simulink model "IEEE118_FULL_seed17_GFOL_RL_percgfor091_PyStable"  (R2023a)
(part 3 of 3)

  Line-132/RConn1 -- BUS-SG-19/RConn1 -- BUS-89/LConn1 -- Line-131/RConn1
  Line-132/RConn2 -- BUS-SG-19/RConn2 -- BUS-89/LConn2 -- Line-131/RConn2
  Line-132/RConn3 -- BUS-SG-19/RConn3 -- BUS-89/LConn3 -- Line-131/RConn3
  BUS-SG-19/LConn1 -- SG-19/RConn1
  BUS-SG-19/LConn2 -- SG-19/RConn2
  BUS-SG-19/LConn3 -- SG-19/RConn3
  Line-133/LConn1 -- BUS-89/RConn1 -- Line-134/LConn1
  Line-133/LConn2 -- BUS-89/RConn2 -- Line-134/LConn2
  Line-133/LConn3 -- BUS-89/RConn3 -- Line-134/LConn3
  Line-133/RConn1 -- BUS-Load-68/LConn1 -- BUS-90/LConn1 -- BUS-SG-20/RConn1
  Line-133/RConn2 -- BUS-Load-68/LConn2 -- BUS-90/LConn2 -- BUS-SG-20/RConn2
  Line-133/RConn3 -- BUS-Load-68/LConn3 -- BUS-90/LConn3 -- BUS-SG-20/RConn3
  BUS-Load-68/RConn1 -- Load-68/LConn1
  BUS-Load-68/RConn2 -- Load-68/LConn2
  BUS-Load-68/RConn3 -- Load-68/LConn3
  BUS-SG-20/LConn1 -- SG-20/RConn1
  BUS-SG-20/LConn2 -- SG-20/RConn2
  BUS-SG-20/LConn3 -- SG-20/RConn3
  BUS-90/RConn1 -- Line-135/LConn1
  BUS-90/RConn2 -- Line-135/LConn2
  BUS-90/RConn3 -- Line-135/LConn3
  Line-135/RConn1 -- BUS-91/LConn1
  Line-135/RConn2 -- BUS-91/LConn2
  Line-135/RConn3 -- BUS-91/LConn3
  BUS-91/RConn1 -- Line-136/LConn1
  BUS-91/RConn2 -- Line-136/LConn2
  BUS-91/RConn3 -- Line-136/LConn3
  BUS-92/LConn1 -- Line-136/RConn1 -- Line-134/RConn1
  BUS-92/LConn2 -- Line-136/RConn2 -- Line-134/RConn2
  BUS-92/LConn3 -- Line-136/RConn3 -- Line-134/RConn3
  BUS-Load-69/LConn1 -- BUS-92/RConn1 -- BUS-SG-21/RConn1 -- BUS-VSC-6/RConn1 -- BUS-VSC-16/RConn1 -- Line-137/LConn1 -- Line-140/LConn1 -- Line-139/LConn1 -- Line-138/LConn1
  BUS-Load-69/LConn2 -- BUS-92/RConn2 -- BUS-SG-21/RConn2 -- BUS-VSC-6/RConn2 -- BUS-VSC-16/RConn2 -- Line-137/LConn2 -- Line-140/LConn2 -- Line-139/LConn2 -- Line-138/LConn2
  BUS-Load-69/LConn3 -- BUS-92/RConn3 -- BUS-SG-21/RConn3 -- BUS-VSC-6/RConn3 -- BUS-VSC-16/RConn3 -- Line-137/LConn3 -- Line-140/LConn3 -- Line-139/LConn3 -- Line-138/LConn3
  BUS-Load-69/RConn1 -- Load-69/LConn1
  BUS-Load-69/RConn2 -- Load-69/LConn2
  BUS-Load-69/RConn3 -- Load-69/LConn3
  BUS-SG-21/LConn1 -- SG-21/RConn1
  BUS-SG-21/LConn2 -- SG-21/RConn2
  BUS-SG-21/LConn3 -- SG-21/RConn3
  BUS-VSC-6/LConn1 -- VSC-6/RConn1
  BUS-VSC-6/LConn2 -- VSC-6/RConn2
  BUS-VSC-6/LConn3 -- VSC-6/RConn3
  BUS-VSC-16/LConn1 -- VSC-16/RConn1
  BUS-VSC-16/LConn2 -- VSC-16/RConn2
  BUS-VSC-16/LConn3 -- VSC-16/RConn3
  BUS-93/LConn1 -- Line-137/RConn1 -- Line-141/LConn1
  BUS-93/LConn2 -- Line-137/RConn2 -- Line-141/LConn2
  BUS-93/LConn3 -- Line-137/RConn3 -- Line-141/LConn3
  BUS-93/RConn1 -- BUS-Load-70/LConn1
  BUS-93/RConn2 -- BUS-Load-70/LConn2
  BUS-93/RConn3 -- BUS-Load-70/LConn3
  BUS-Load-70/RConn1 -- Load-70/LConn1
  BUS-Load-70/RConn2 -- Load-70/LConn2
  BUS-Load-70/RConn3 -- Load-70/LConn3
  Line-141/RConn1 -- BUS-Load-71/LConn1 -- Line-142/LConn1 -- BUS-94/RConn1 -- Line-144/LConn1
  Line-141/RConn2 -- BUS-Load-71/LConn2 -- Line-142/LConn2 -- BUS-94/RConn2 -- Line-144/LConn2
  Line-141/RConn3 -- BUS-Load-71/LConn3 -- Line-142/LConn3 -- BUS-94/RConn3 -- Line-144/LConn3
  BUS-Load-71/RConn1 -- Load-71/LConn1
  BUS-Load-71/RConn2 -- Load-71/LConn2
  BUS-Load-71/RConn3 -- Load-71/LConn3
  BUS-95/LConn1 -- Line-142/RConn1 -- Line-145/LConn1
  BUS-95/LConn2 -- Line-142/RConn2 -- Line-145/LConn2
  BUS-95/LConn3 -- Line-142/RConn3 -- Line-145/LConn3
  BUS-95/RConn1 -- BUS-Load-72/LConn1
  BUS-95/RConn2 -- BUS-Load-72/LConn2
  BUS-95/RConn3 -- BUS-Load-72/LConn3
  BUS-Load-72/RConn1 -- Load-72/LConn1
  BUS-Load-72/RConn2 -- Load-72/LConn2
  BUS-Load-72/RConn3 -- Load-72/LConn3
  Line-143/LConn1 -- BUS-94/LConn1 -- Line-138/RConn1
  Line-143/LConn2 -- BUS-94/LConn2 -- Line-138/RConn2
  Line-143/LConn3 -- BUS-94/LConn3 -- Line-138/RConn3
  Line-144/RConn1 -- BUS-Load-76/LConn1 -- BUS-SG-22/RConn1 -- BUS-VSC-7/RConn1 -- Line-149/LConn1 -- Line-139/RConn1 -- Line-147/RConn1 -- BUS-100/LConn1 -- Line-148/RConn1
  Line-144/RConn2 -- BUS-Load-76/LConn2 -- BUS-SG-22/RConn2 -- BUS-VSC-7/RConn2 -- Line-149/LConn2 -- Line-139/RConn2 -- Line-147/RConn2 -- BUS-100/LConn2 -- Line-148/RConn2
  Line-144/RConn3 -- BUS-Load-76/LConn3 -- BUS-SG-22/RConn3 -- BUS-VSC-7/RConn3 -- Line-149/LConn3 -- Line-139/RConn3 -- Line-147/RConn3 -- BUS-100/LConn3 -- Line-148/RConn3
  BUS-Load-76/RConn1 -- Load-76/LConn1
  BUS-Load-76/RConn2 -- Load-76/LConn2
  BUS-Load-76/RConn3 -- Load-76/LConn3
  BUS-SG-22/LConn1 -- SG-22/RConn1
  BUS-SG-22/LConn2 -- SG-22/RConn2
  BUS-SG-22/LConn3 -- SG-22/RConn3
  BUS-VSC-7/LConn1 -- VSC-7/RConn1
  BUS-VSC-7/LConn2 -- VSC-7/RConn2
  BUS-VSC-7/LConn3 -- VSC-7/RConn3
  BUS-VSC-17/RConn1 -- BUS-100/RConn1 -- Line-150/LConn1 -- Line-152/LConn1 -- Line-151/LConn1
  BUS-VSC-17/RConn2 -- BUS-100/RConn2 -- Line-150/LConn2 -- Line-152/LConn2 -- Line-151/LConn2
  BUS-VSC-17/RConn3 -- BUS-100/RConn3 -- Line-150/LConn3 -- Line-152/LConn3 -- Line-151/LConn3
  BUS-VSC-17/LConn1 -- VSC-17/RConn1
  BUS-VSC-17/LConn2 -- VSC-17/RConn2
  BUS-VSC-17/LConn3 -- VSC-17/RConn3
  BUS-101/RConn1 -- Line-149/RConn1 -- Line-153/LConn1
  BUS-101/RConn2 -- Line-149/RConn2 -- Line-153/LConn2
  BUS-101/RConn3 -- Line-149/RConn3 -- Line-153/LConn3
  BUS-101/LConn1 -- BUS-Load-77/LConn1
  BUS-101/LConn2 -- BUS-Load-77/LConn2
  BUS-101/LConn3 -- BUS-Load-77/LConn3
  BUS-Load-77/RConn1 -- Load-77/LConn1
  BUS-Load-77/RConn2 -- Load-77/LConn2
  BUS-Load-77/RConn3 -- Load-77/LConn3
  BUS-102/LConn1 -- Line-153/RConn1 -- Line-140/RConn1
  BUS-102/LConn2 -- Line-153/RConn2 -- Line-140/RConn2
  BUS-102/LConn3 -- Line-153/RConn3 -- Line-140/RConn3
  BUS-102/RConn1 -- BUS-Load-78/LConn1
  BUS-102/RConn2 -- BUS-Load-78/LConn2
  BUS-102/RConn3 -- BUS-Load-78/LConn3
  BUS-Load-78/RConn1 -- Load-78/LConn1
  BUS-Load-78/RConn2 -- Load-78/LConn2
  BUS-Load-78/RConn3 -- Load-78/LConn3
  Line-150/RConn1 -- Line-154/LConn1 -- BUS-103/LConn1 -- Line-155/LConn1
  Line-150/RConn2 -- Line-154/LConn2 -- BUS-103/LConn2 -- Line-155/LConn2
  Line-150/RConn3 -- Line-154/LConn3 -- BUS-103/LConn3 -- Line-155/LConn3
  BUS-Load-79/LConn1 -- BUS-103/RConn1 -- Line-156/LConn1
  BUS-Load-79/LConn2 -- BUS-103/RConn2 -- Line-156/LConn2
  BUS-Load-79/LConn3 -- BUS-103/RConn3 -- Line-156/LConn3
  BUS-Load-79/RConn1 -- Load-79/LConn1
  BUS-Load-79/RConn2 -- Load-79/LConn2
  BUS-Load-79/RConn3 -- Load-79/LConn3
  Line-154/RConn1 -- BUS-Load-80/LConn1 -- BUS-104/RConn1 -- Line-157/LConn1
  Line-154/RConn2 -- BUS-Load-80/LConn2 -- BUS-104/RConn2 -- Line-157/LConn2
  Line-154/RConn3 -- BUS-Load-80/LConn3 -- BUS-104/RConn3 -- Line-157/LConn3
  BUS-Load-80/RConn1 -- Load-80/LConn1
  BUS-Load-80/RConn2 -- Load-80/LConn2
  BUS-Load-80/RConn3 -- Load-80/LConn3
  Line-157/RConn1 -- BUS-VSC-18/RConn1 -- Line-158/LConn1 -- BUS-105/LConn1 -- Line-159/LConn1
  Line-157/RConn2 -- BUS-VSC-18/RConn2 -- Line-158/LConn2 -- BUS-105/LConn2 -- Line-159/LConn2
  Line-157/RConn3 -- BUS-VSC-18/RConn3 -- Line-158/LConn3 -- BUS-105/LConn3 -- Line-159/LConn3
  BUS-Load-81/LConn1 -- BUS-105/RConn1 -- BUS-SG-23/RConn1 -- BUS-VSC-8/RConn1 -- Line-160/LConn1 -- Line-155/RConn1
  BUS-Load-81/LConn2 -- BUS-105/RConn2 -- BUS-SG-23/RConn2 -- BUS-VSC-8/RConn2 -- Line-160/LConn2 -- Line-155/RConn2
  BUS-Load-81/LConn3 -- BUS-105/RConn3 -- BUS-SG-23/RConn3 -- BUS-VSC-8/RConn3 -- Line-160/LConn3 -- Line-155/RConn3
  BUS-Load-81/RConn1 -- Load-81/LConn1
  BUS-Load-81/RConn2 -- Load-81/LConn2
  BUS-Load-81/RConn3 -- Load-81/LConn3
  BUS-SG-23/LConn1 -- SG-23/RConn1
  BUS-SG-23/LConn2 -- SG-23/RConn2
  BUS-SG-23/LConn3 -- SG-23/RConn3
  BUS-VSC-8/LConn1 -- VSC-8/RConn1
  BUS-VSC-8/LConn2 -- VSC-8/RConn2
  BUS-VSC-8/LConn3 -- VSC-8/RConn3
  BUS-VSC-18/LConn1 -- VSC-18/RConn1
  BUS-VSC-18/LConn2 -- VSC-18/RConn2
  BUS-VSC-18/LConn3 -- VSC-18/RConn3
  BUS-106/RConn1 -- Line-158/RConn1 -- Line-161/LConn1
  BUS-106/RConn2 -- Line-158/RConn2 -- Line-161/LConn2
  BUS-106/RConn3 -- Line-158/RConn3 -- Line-161/LConn3
  BUS-Load-82/LConn1 -- BUS-106/LConn1 -- Line-152/RConn1
  BUS-Load-82/LConn2 -- BUS-106/LConn2 -- Line-152/RConn2
  BUS-Load-82/LConn3 -- BUS-106/LConn3 -- Line-152/RConn3
  BUS-Load-82/RConn1 -- Load-82/LConn1
  BUS-Load-82/RConn2 -- Load-82/LConn2
  BUS-Load-82/RConn3 -- Load-82/LConn3
  Line-161/RConn1 -- BUS-Load-83/LConn1 -- BUS-107/LConn1 -- BUS-SG-24/RConn1
  Line-161/RConn2 -- BUS-Load-83/LConn2 -- BUS-107/LConn2 -- BUS-SG-24/RConn2
  Line-161/RConn3 -- BUS-Load-83/LConn3 -- BUS-107/LConn3 -- BUS-SG-24/RConn3
  BUS-Load-83/RConn1 -- Load-83/LConn1
  BUS-Load-83/RConn2 -- Load-83/LConn2
  BUS-Load-83/RConn3 -- Load-83/LConn3
  BUS-SG-24/LConn1 -- SG-24/RConn1
  BUS-SG-24/LConn2 -- SG-24/RConn2
  BUS-SG-24/LConn3 -- SG-24/RConn3
  Line-159/RConn1 -- BUS-107/RConn1
  Line-159/RConn2 -- BUS-107/RConn2
  Line-159/RConn3 -- BUS-107/RConn3
  Line-160/RConn1 -- BUS-108/LConn1
  Line-160/RConn2 -- BUS-108/LConn2
  Line-160/RConn3 -- BUS-108/LConn3
  BUS-Load-84/LConn1 -- BUS-108/RConn1 -- Line-162/LConn1
  BUS-Load-84/LConn2 -- BUS-108/RConn2 -- Line-162/LConn2
  BUS-Load-84/LConn3 -- BUS-108/RConn3 -- Line-162/LConn3
  BUS-Load-84/RConn1 -- Load-84/LConn1
  BUS-Load-84/RConn2 -- Load-84/LConn2
  BUS-Load-84/RConn3 -- Load-84/LConn3
  Line-162/RConn1 -- BUS-109/LConn1
  Line-162/RConn2 -- BUS-109/LConn2
  Line-162/RConn3 -- BUS-109/LConn3
  BUS-Load-85/LConn1 -- BUS-109/RConn1 -- Line-163/LConn1
  BUS-Load-85/LConn2 -- BUS-109/RConn2 -- Line-163/LConn2
  BUS-Load-85/LConn3 -- BUS-109/RConn3 -- Line-163/LConn3
  BUS-Load-85/RConn1 -- Load-85/LConn1
  BUS-Load-85/RConn2 -- Load-85/LConn2
  BUS-Load-85/RConn3 -- Load-85/LConn3
  BUS-110/LConn1 -- Line-163/RConn1 -- Line-156/RConn1
  BUS-110/LConn2 -- Line-163/RConn2 -- Line-156/RConn2
  BUS-110/LConn3 -- Line-163/RConn3 -- Line-156/RConn3
  BUS-Load-86/LConn1 -- BUS-110/RConn1 -- BUS-VSC-9/RConn1 -- BUS-VSC-19/RConn1 -- Line-164/LConn1
  BUS-Load-86/LConn2 -- BUS-110/RConn2 -- BUS-VSC-9/RConn2 -- BUS-VSC-19/RConn2 -- Line-164/LConn2
  BUS-Load-86/LConn3 -- BUS-110/RConn3 -- BUS-VSC-9/RConn3 -- BUS-VSC-19/RConn3 -- Line-164/LConn3
  BUS-Load-86/RConn1 -- Load-86/LConn1
  BUS-Load-86/RConn2 -- Load-86/LConn2
  BUS-Load-86/RConn3 -- Load-86/LConn3
  BUS-VSC-9/LConn1 -- VSC-9/RConn1
  BUS-VSC-9/LConn2 -- VSC-9/RConn2
  BUS-VSC-9/LConn3 -- VSC-9/RConn3
  BUS-VSC-19/LConn1 -- VSC-19/RConn1
  BUS-VSC-19/LConn2 -- VSC-19/RConn2
  BUS-VSC-19/LConn3 -- VSC-19/RConn3
  Line-164/RConn1 -- BUS-112/LConn1
  Line-164/RConn2 -- BUS-112/LConn2
  Line-164/RConn3 -- BUS-112/LConn3
  BUS-Load-87/LConn1 -- BUS-112/RConn1 -- BUS-SG-25/RConn1 -- BUS-VSC-10/RConn1 -- BUS-VSC-20/RConn1
  BUS-Load-87/LConn2 -- BUS-112/RConn2 -- BUS-SG-25/RConn2 -- BUS-VSC-10/RConn2 -- BUS-VSC-20/RConn2
  BUS-Load-87/LConn3 -- BUS-112/RConn3 -- BUS-SG-25/RConn3 -- BUS-VSC-10/RConn3 -- BUS-VSC-20/RConn3
  BUS-Load-87/RConn1 -- Load-87/LConn1
  BUS-Load-87/RConn2 -- Load-87/LConn2
  BUS-Load-87/RConn3 -- Load-87/LConn3
  BUS-SG-25/LConn1 -- SG-25/RConn1
  BUS-SG-25/LConn2 -- SG-25/RConn2
  BUS-SG-25/LConn3 -- SG-25/RConn3
  BUS-VSC-10/LConn1 -- VSC-10/RConn1
  BUS-VSC-10/LConn2 -- VSC-10/RConn2
  BUS-VSC-10/LConn3 -- VSC-10/RConn3
  BUS-VSC-20/LConn1 -- VSC-20/RConn1
  BUS-VSC-20/LConn2 -- VSC-20/RConn2
  BUS-VSC-20/LConn3 -- VSC-20/RConn3
  Line-151/RConn1 -- BUS-104/LConn1
  Line-151/RConn2 -- BUS-104/LConn2
  Line-151/RConn3 -- BUS-104/LConn3
  BUS-98/RConn1 -- Line-147/LConn1
  BUS-98/RConn2 -- Line-147/LConn2
  BUS-98/RConn3 -- Line-147/LConn3
  BUS-Load-75/LConn1 -- BUS-98/LConn1 -- Line-122/RConn1
  BUS-Load-75/LConn2 -- BUS-98/LConn2 -- Line-122/RConn2
  BUS-Load-75/LConn3 -- BUS-98/LConn3 -- Line-122/RConn3
  BUS-Load-75/RConn1 -- Load-75/LConn1
  BUS-Load-75/RConn2 -- Load-75/LConn2
  BUS-Load-75/RConn3 -- Load-75/LConn3
  BUS-99/RConn1 -- Line-148/LConn1
  BUS-99/RConn2 -- Line-148/LConn2
  BUS-99/RConn3 -- Line-148/LConn3
  Line-123/RConn1 -- BUS-99/LConn1
  Line-123/RConn2 -- BUS-99/LConn2
  Line-123/RConn3 -- BUS-99/LConn3
  Line-117/LConn1 -- BUS-77/LConn1 -- BUS-Load-58/LConn1 -- BUS-SG-16/RConn1 -- Line-115/LConn1 -- Line-113/RConn1
  Line-117/LConn2 -- BUS-77/LConn2 -- BUS-Load-58/LConn2 -- BUS-SG-16/RConn2 -- Line-115/LConn2 -- Line-113/RConn2
  Line-117/LConn3 -- BUS-77/LConn3 -- BUS-Load-58/LConn3 -- BUS-SG-16/RConn3 -- Line-115/LConn3 -- Line-113/RConn3
  BUS-Load-58/RConn1 -- Load-58/LConn1
  BUS-Load-58/RConn2 -- Load-58/LConn2
  BUS-Load-58/RConn3 -- Load-58/LConn3
  BUS-SG-16/LConn1 -- SG-16/RConn1
  BUS-SG-16/LConn2 -- SG-16/RConn2
  BUS-SG-16/LConn3 -- SG-16/RConn3
  BUS-78/RConn1 -- Line-115/RConn1 -- Line-118/LConn1
  BUS-78/RConn2 -- Line-115/RConn2 -- Line-118/LConn2
  BUS-78/RConn3 -- Line-115/RConn3 -- Line-118/LConn3
  BUS-78/LConn1 -- BUS-Load-59/LConn1
  BUS-78/LConn2 -- BUS-Load-59/LConn2
  BUS-78/LConn3 -- BUS-Load-59/LConn3
  BUS-Load-59/RConn1 -- Load-59/LConn1
  BUS-Load-59/RConn2 -- Load-59/LConn2
  BUS-Load-59/RConn3 -- Load-59/LConn3
  BUS-79/LConn1 -- Line-118/RConn1 -- BUS-Load-60/LConn1
  BUS-79/LConn2 -- Line-118/RConn2 -- BUS-Load-60/LConn2
  BUS-79/LConn3 -- Line-118/RConn3 -- BUS-Load-60/LConn3
  BUS-Load-60/RConn1 -- Load-60/LConn1
  BUS-Load-60/RConn2 -- Load-60/LConn2
  BUS-Load-60/RConn3 -- Load-60/LConn3
  BUS-79/RConn1 -- Line-119/LConn1
  BUS-79/RConn2 -- Line-119/LConn2
  BUS-79/RConn3 -- Line-119/LConn3
  Line-116/LConn1 -- BUS-77/RConn1 -- Line-104/RConn1 -- Line-111/RConn1
  Line-116/LConn2 -- BUS-77/RConn2 -- Line-104/RConn2 -- Line-111/RConn2
  Line-116/LConn3 -- BUS-77/RConn3 -- Line-104/RConn3 -- Line-111/RConn3
  Line-104/LConn1 -- BUS-69/LConn1 -- Line-103/LConn1
  Line-104/LConn2 -- BUS-69/LConn2 -- Line-103/LConn2
  Line-104/LConn3 -- BUS-69/LConn3 -- Line-103/LConn3
  Line-102/LConn1 -- BUS-69/RConn1 -- Line-76/RConn1 -- Line-70/RConn1 -- Line-173/RConn1
  Line-102/LConn2 -- BUS-69/RConn2 -- Line-76/RConn2 -- Line-70/RConn2 -- Line-173/RConn2
  Line-102/LConn3 -- BUS-69/RConn3 -- Line-76/RConn3 -- Line-70/RConn3 -- Line-173/RConn3
  Line-102/RConn1 -- Line-105/LConn1 -- Line-106/LConn1 -- BUS-70/LConn1 -- Line-107/LConn1
  Line-102/RConn2 -- Line-105/LConn2 -- Line-106/LConn2 -- BUS-70/LConn2 -- Line-107/LConn2
  Line-102/RConn3 -- Line-105/LConn3 -- Line-106/LConn3 -- BUS-70/LConn3 -- Line-107/LConn3
  BUS-Load-54/LConn1 -- BUS-70/RConn1 -- BUS-SG-12/RConn1 -- Line-36/RConn1
  BUS-Load-54/LConn2 -- BUS-70/RConn2 -- BUS-SG-12/RConn2 -- Line-36/RConn2
  BUS-Load-54/LConn3 -- BUS-70/RConn3 -- BUS-SG-12/RConn3 -- Line-36/RConn3
  BUS-Load-54/RConn1 -- Load-54/LConn1
  BUS-Load-54/RConn2 -- Load-54/LConn2
  BUS-Load-54/RConn3 -- Load-54/LConn3
  BUS-SG-12/LConn1 -- SG-12/RConn1
  BUS-SG-12/LConn2 -- SG-12/RConn2
  BUS-SG-12/LConn3 -- SG-12/RConn3
  BUS-71/RConn1 -- Line-105/RConn1 -- Line-108/LConn1
  BUS-71/RConn2 -- Line-105/RConn2 -- Line-108/LConn2
  BUS-71/RConn3 -- Line-105/RConn3 -- Line-108/LConn3
  Line-108/RConn1 -- BUS-72/LConn1
  Line-108/RConn2 -- BUS-72/LConn2
  Line-108/RConn3 -- BUS-72/LConn3
  BUS-SG-13/RConn1 -- BUS-72/RConn1 -- Line-37/RConn1
  BUS-SG-13/RConn2 -- BUS-72/RConn2 -- Line-37/RConn2
  BUS-SG-13/RConn3 -- BUS-72/RConn3 -- Line-37/RConn3
  BUS-SG-13/LConn1 -- SG-13/RConn1
  BUS-SG-13/LConn2 -- SG-13/RConn2
  BUS-SG-13/LConn3 -- SG-13/RConn3
  Line-37/LConn1 -- BUS-24/LConn1 -- Line-36/LConn1
  Line-37/LConn2 -- BUS-24/LConn2 -- Line-36/LConn2
  Line-37/LConn3 -- BUS-24/LConn3 -- Line-36/LConn3
  Line-33/LConn1 -- BUS-23/LConn1 -- BUS-Load-19/LConn1
  Line-33/LConn2 -- BUS-23/LConn2 -- BUS-Load-19/LConn2
  Line-33/LConn3 -- BUS-23/LConn3 -- BUS-Load-19/LConn3
  Line-33/RConn1 -- BUS-24/RConn1
  Line-33/RConn2 -- BUS-24/RConn2
  Line-33/RConn3 -- BUS-24/RConn3
  BUS-Load-19/RConn1 -- Load-19/LConn1
  BUS-Load-19/RConn2 -- Load-19/LConn2
  BUS-Load-19/RConn3 -- Load-19/LConn3
  Line-34/LConn1 -- BUS-23/RConn1 -- Line-32/RConn1 -- Line-35/LConn1
  Line-34/LConn2 -- BUS-23/RConn2 -- Line-32/RConn2 -- Line-35/LConn2
  Line-34/LConn3 -- BUS-23/RConn3 -- Line-32/RConn3 -- Line-35/LConn3
  Line-34/RConn1 -- BUS-25/LConn1
  Line-34/RConn2 -- BUS-25/LConn2
  Line-34/RConn3 -- BUS-25/LConn3
  Line-38/LConn1 -- BUS-25/RConn1 -- Line-168/LConn1
  Line-38/LConn2 -- BUS-25/RConn2 -- Line-168/LConn2
  Line-38/LConn3 -- BUS-25/RConn3 -- Line-168/LConn3
  Line-38/RConn1 -- BUS-Load-20/LConn1 -- BUS-27/LConn1 -- Line-41/LConn1
  Line-38/RConn2 -- BUS-Load-20/LConn2 -- BUS-27/LConn2 -- Line-41/LConn2
  Line-38/RConn3 -- BUS-Load-20/LConn3 -- BUS-27/LConn3 -- Line-41/LConn3
  BUS-Load-20/RConn1 -- Load-20/LConn1
  BUS-Load-20/RConn2 -- Load-20/LConn2
  BUS-Load-20/RConn3 -- Load-20/LConn3
  Line-40/LConn1 -- BUS-27/RConn1 -- Line-42/LConn1
  Line-40/LConn2 -- BUS-27/RConn2 -- Line-42/LConn2
  Line-40/LConn3 -- BUS-27/RConn3 -- Line-42/LConn3
  Line-40/RConn1 -- BUS-28/LConn1
  Line-40/RConn2 -- BUS-28/LConn2
  Line-40/RConn3 -- BUS-28/LConn3
  BUS-Load-21/LConn1 -- BUS-28/RConn1 -- Line-43/LConn1
  BUS-Load-21/LConn2 -- BUS-28/RConn2 -- Line-43/LConn2
  BUS-Load-21/LConn3 -- BUS-28/RConn3 -- Line-43/LConn3
  BUS-Load-21/RConn1 -- Load-21/LConn1
  BUS-Load-21/RConn2 -- Load-21/LConn2
  BUS-Load-21/RConn3 -- Load-21/LConn3
  BUS-29/LConn1 -- Line-43/RConn1 -- Line-44/LConn1
  BUS-29/LConn2 -- Line-43/RConn2 -- Line-44/LConn2
  BUS-29/LConn3 -- Line-43/RConn3 -- Line-44/LConn3
  BUS-29/RConn1 -- BUS-Load-22/LConn1
  BUS-29/RConn2 -- BUS-Load-22/LConn2
  BUS-29/RConn3 -- BUS-Load-22/LConn3
  BUS-Load-22/RConn1 -- Load-22/LConn1
  BUS-Load-22/RConn2 -- Load-22/LConn2
  BUS-Load-22/RConn3 -- Load-22/LConn3
  Line-44/RConn1 -- BUS-VSC-2/RConn1 -- BUS-VSC-12/RConn1 -- BUS-31/RConn1 -- Line-25/RConn1
  Line-44/RConn2 -- BUS-VSC-2/RConn2 -- BUS-VSC-12/RConn2 -- BUS-31/RConn2 -- Line-25/RConn2
  Line-44/RConn3 -- BUS-VSC-2/RConn3 -- BUS-VSC-12/RConn3 -- BUS-31/RConn3 -- Line-25/RConn3
  BUS-Load-23/LConn1 -- BUS-31/LConn1 -- Line-46/LConn1
  BUS-Load-23/LConn2 -- BUS-31/LConn2 -- Line-46/LConn2
  BUS-Load-23/LConn3 -- BUS-31/LConn3 -- Line-46/LConn3
  BUS-Load-23/RConn1 -- Load-23/LConn1
  BUS-Load-23/RConn2 -- Load-23/LConn2
  BUS-Load-23/RConn3 -- Load-23/LConn3
  BUS-VSC-2/LConn1 -- VSC-2/RConn1
  BUS-VSC-2/LConn2 -- VSC-2/RConn2
  BUS-VSC-2/LConn3 -- VSC-2/RConn3
  BUS-VSC-12/LConn1 -- VSC-12/RConn1
  BUS-VSC-12/LConn2 -- VSC-12/RConn2
  BUS-VSC-12/LConn3 -- VSC-12/RConn3
  Line-46/RConn1 -- BUS-VSC-3/RConn1 -- Line-47/LConn1 -- Line-48/LConn1 -- BUS-32/RConn1 -- Line-41/RConn1
  Line-46/RConn2 -- BUS-VSC-3/RConn2 -- Line-47/LConn2 -- Line-48/LConn2 -- BUS-32/RConn2 -- Line-41/RConn2
  Line-46/RConn3 -- BUS-VSC-3/RConn3 -- Line-47/LConn3 -- Line-48/LConn3 -- BUS-32/RConn3 -- Line-41/RConn3
  BUS-Load-24/LConn1 -- BUS-32/LConn1 -- BUS-SG-3/RConn1 -- BUS-VSC-13/RConn1 -- Line-35/RConn1
  BUS-Load-24/LConn2 -- BUS-32/LConn2 -- BUS-SG-3/RConn2 -- BUS-VSC-13/RConn2 -- Line-35/RConn2
  BUS-Load-24/LConn3 -- BUS-32/LConn3 -- BUS-SG-3/RConn3 -- BUS-VSC-13/RConn3 -- Line-35/RConn3
  BUS-Load-24/RConn1 -- Load-24/LConn1
  BUS-Load-24/RConn2 -- Load-24/LConn2
  BUS-Load-24/RConn3 -- Load-24/LConn3
  BUS-SG-3/LConn1 -- SG-3/RConn1
  BUS-SG-3/LConn2 -- SG-3/RConn2
  BUS-SG-3/LConn3 -- SG-3/RConn3
  BUS-VSC-3/LConn1 -- VSC-3/RConn1
  BUS-VSC-3/LConn2 -- VSC-3/RConn2
  BUS-VSC-3/LConn3 -- VSC-3/RConn3
  BUS-VSC-13/LConn1 -- VSC-13/RConn1
  BUS-VSC-13/LConn2 -- VSC-13/RConn2
  BUS-VSC-13/LConn3 -- VSC-13/RConn3
  BUS-113/LConn1 -- Line-47/RConn1 -- BUS-SG-26/RConn1
  BUS-113/LConn2 -- Line-47/RConn2 -- BUS-SG-26/RConn2
  BUS-113/LConn3 -- Line-47/RConn3 -- BUS-SG-26/RConn3
  BUS-SG-26/LConn1 -- SG-26/RConn1
  BUS-SG-26/LConn2 -- SG-26/RConn2
  BUS-SG-26/LConn3 -- SG-26/RConn3
  Line-26/LConn1 -- BUS-17/LConn1 -- Line-167/LConn1 -- Line-25/LConn1
  Line-26/LConn2 -- BUS-17/LConn2 -- Line-167/LConn2 -- Line-25/LConn2
  Line-26/LConn3 -- BUS-17/LConn3 -- Line-167/LConn3 -- Line-25/LConn3
  Line-26/RConn1 -- BUS-113/RConn1
  Line-26/RConn2 -- BUS-113/RConn2
  Line-26/RConn3 -- BUS-113/RConn3
  BUS-Load-13/LConn1 -- BUS-17/RConn1 -- Line-24/LConn1 -- Line-20/RConn1 -- Line-23/RConn1
  BUS-Load-13/LConn2 -- BUS-17/RConn2 -- Line-24/LConn2 -- Line-20/RConn2 -- Line-23/RConn2
  BUS-Load-13/LConn3 -- BUS-17/RConn3 -- Line-24/LConn3 -- Line-20/RConn3 -- Line-23/RConn3
  BUS-Load-13/RConn1 -- Load-13/LConn1
  BUS-Load-13/RConn2 -- Load-13/LConn2
  BUS-Load-13/RConn3 -- Load-13/LConn3
  BUS-18/LConn1 -- Line-24/RConn1 -- BUS-Load-14/LConn1
  BUS-18/LConn2 -- Line-24/RConn2 -- BUS-Load-14/LConn2
  BUS-18/LConn3 -- Line-24/RConn3 -- BUS-Load-14/LConn3
  BUS-Load-14/RConn1 -- Load-14/LConn1
  BUS-Load-14/RConn2 -- Load-14/LConn2
  BUS-Load-14/RConn3 -- Load-14/LConn3
  BUS-18/RConn1 -- Line-27/LConn1
  BUS-18/RConn2 -- Line-27/LConn2
  BUS-18/RConn3 -- Line-27/LConn3
  Line-27/RConn1 -- Line-28/LConn1 -- BUS-19/LConn1 -- Line-29/LConn1
  Line-27/RConn2 -- Line-28/LConn2 -- BUS-19/LConn2 -- Line-29/LConn2
  Line-27/RConn3 -- Line-28/LConn3 -- BUS-19/LConn3 -- Line-29/LConn3
  BUS-Load-15/LConn1 -- BUS-19/RConn1 -- BUS-SG-2/RConn1 -- BUS-VSC-1/RConn1 -- BUS-VSC-11/RConn1 -- Line-21/RConn1
  BUS-Load-15/LConn2 -- BUS-19/RConn2 -- BUS-SG-2/RConn2 -- BUS-VSC-1/RConn2 -- BUS-VSC-11/RConn2 -- Line-21/RConn2
  BUS-Load-15/LConn3 -- BUS-19/RConn3 -- BUS-SG-2/RConn3 -- BUS-VSC-1/RConn3 -- BUS-VSC-11/RConn3 -- Line-21/RConn3
  BUS-Load-15/RConn1 -- Load-15/LConn1
  BUS-Load-15/RConn2 -- Load-15/LConn2
  BUS-Load-15/RConn3 -- Load-15/LConn3
  BUS-SG-2/LConn1 -- SG-2/RConn1
  BUS-SG-2/LConn2 -- SG-2/RConn2
  BUS-SG-2/LConn3 -- SG-2/RConn3
  BUS-VSC-1/LConn1 -- VSC-1/RConn1
  BUS-VSC-1/LConn2 -- VSC-1/RConn2
  BUS-VSC-1/LConn3 -- VSC-1/RConn3
  BUS-VSC-11/LConn1 -- VSC-11/RConn1
  BUS-VSC-11/LConn2 -- VSC-11/RConn2
  BUS-VSC-11/LConn3 -- VSC-11/RConn3
  BUS-20/RConn1 -- Line-28/RConn1 -- BUS-Load-16/LConn1
  BUS-20/RConn2 -- Line-28/RConn2 -- BUS-Load-16/LConn2
  BUS-20/RConn3 -- Line-28/RConn3 -- BUS-Load-16/LConn3
  BUS-Load-16/RConn1 -- Load-16/LConn1
  BUS-Load-16/RConn2 -- Load-16/LConn2
  BUS-Load-16/RConn3 -- Load-16/LConn3
  BUS-20/LConn1 -- Line-30/LConn1
  BUS-20/LConn2 -- Line-30/LConn2
  BUS-20/LConn3 -- Line-30/LConn3
  BUS-21/RConn1 -- Line-30/RConn1 -- BUS-Load-17/LConn1
  BUS-21/RConn2 -- Line-30/RConn2 -- BUS-Load-17/LConn2
  BUS-21/RConn3 -- Line-30/RConn3 -- BUS-Load-17/LConn3
  BUS-Load-17/RConn1 -- Load-17/LConn1
  BUS-Load-17/RConn2 -- Load-17/LConn2
  BUS-Load-17/RConn3 -- Load-17/LConn3
  BUS-21/LConn1 -- Line-31/LConn1
  BUS-21/LConn2 -- Line-31/LConn2
  BUS-21/LConn3 -- Line-31/LConn3
  Line-31/RConn1 -- BUS-22/RConn1
  Line-31/RConn2 -- BUS-22/RConn2
  Line-31/RConn3 -- BUS-22/RConn3
  BUS-Load-18/LConn1 -- BUS-22/LConn1 -- Line-32/LConn1
  BUS-Load-18/LConn2 -- BUS-22/LConn2 -- Line-32/LConn2
  BUS-Load-18/LConn3 -- BUS-22/LConn3 -- Line-32/LConn3
  BUS-Load-18/RConn1 -- Load-18/LConn1
  BUS-Load-18/RConn2 -- Load-18/LConn2
  BUS-Load-18/RConn3 -- Load-18/LConn3
  Line-29/RConn1 -- BUS-Load-26/LConn1 -- BUS-SG-4/RConn1 -- BUS-34/RConn1 -- Line-50/LConn1
  Line-29/RConn2 -- BUS-Load-26/LConn2 -- BUS-SG-4/RConn2 -- BUS-34/RConn2 -- Line-50/LConn2
  Line-29/RConn3 -- BUS-Load-26/LConn3 -- BUS-SG-4/RConn3 -- BUS-34/RConn3 -- Line-50/LConn3
  BUS-Load-26/RConn1 -- Load-26/LConn1
  BUS-Load-26/RConn2 -- Load-26/LConn2
  BUS-Load-26/RConn3 -- Load-26/LConn3
  BUS-SG-4/LConn1 -- SG-4/RConn1
  BUS-SG-4/LConn2 -- SG-4/RConn2
  BUS-SG-4/LConn3 -- SG-4/RConn3
  BUS-36/LConn1 -- Line-50/RConn1 -- Line-53/RConn1
  BUS-36/LConn2 -- Line-50/RConn2 -- Line-53/RConn2
  BUS-36/LConn3 -- Line-50/RConn3 -- Line-53/RConn3
  BUS-Load-28/LConn1 -- BUS-36/RConn1 -- BUS-SG-5/RConn1
  BUS-Load-28/LConn2 -- BUS-36/RConn2 -- BUS-SG-5/RConn2
  BUS-Load-28/LConn3 -- BUS-36/RConn3 -- BUS-SG-5/RConn3
  BUS-Load-28/RConn1 -- Load-28/LConn1
  BUS-Load-28/RConn2 -- Load-28/LConn2
  BUS-Load-28/RConn3 -- Load-28/LConn3
  BUS-SG-5/LConn1 -- SG-5/RConn1
  BUS-SG-5/LConn2 -- SG-5/RConn2
  BUS-SG-5/LConn3 -- SG-5/RConn3
  Line-53/LConn1 -- BUS-35/RConn1 -- BUS-Load-27/LConn1
  Line-53/LConn2 -- BUS-35/RConn2 -- BUS-Load-27/LConn2
  Line-53/LConn3 -- BUS-35/RConn3 -- BUS-Load-27/LConn3
  BUS-Load-27/RConn1 -- Load-27/LConn1
  BUS-Load-27/RConn2 -- Load-27/LConn2
  BUS-Load-27/RConn3 -- Load-27/LConn3
  BUS-35/LConn1 -- Line-54/LConn1
  BUS-35/LConn2 -- Line-54/LConn2
  BUS-35/LConn3 -- Line-54/LConn3
  Line-54/RConn1 -- BUS-Load-29/LConn1 -- Line-49/RConn1 -- BUS-37/RConn1 -- Line-51/RConn1
  Line-54/RConn2 -- BUS-Load-29/LConn2 -- Line-49/RConn2 -- BUS-37/RConn2 -- Line-51/RConn2
  Line-54/RConn3 -- BUS-Load-29/LConn3 -- Line-49/RConn3 -- BUS-37/RConn3 -- Line-51/RConn3
  BUS-Load-29/RConn1 -- Load-29/LConn1
  BUS-Load-29/RConn2 -- Load-29/LConn2
  BUS-Load-29/RConn3 -- Load-29/LConn3
  Line-55/LConn1 -- BUS-37/LConn1 -- Line-56/LConn1 -- Line-169/LConn1
  Line-55/LConn2 -- BUS-37/LConn2 -- Line-56/LConn2 -- Line-169/LConn2
  Line-55/LConn3 -- BUS-37/LConn3 -- Line-56/LConn3 -- Line-169/LConn3
  Line-55/RConn1 -- BUS-39/RConn1
  Line-55/RConn2 -- BUS-39/RConn2
  Line-55/RConn3 -- BUS-39/RConn3
  BUS-39/LConn1 -- Line-58/LConn1
  BUS-39/LConn2 -- Line-58/LConn2
  BUS-39/LConn3 -- Line-58/LConn3
  Line-58/RConn1 -- BUS-Load-30/LConn1 -- BUS-SG-6/RConn1 -- BUS-40/RConn1 -- Line-56/RConn1
  Line-58/RConn2 -- BUS-Load-30/LConn2 -- BUS-SG-6/RConn2 -- BUS-40/RConn2 -- Line-56/RConn2
  Line-58/RConn3 -- BUS-Load-30/LConn3 -- BUS-SG-6/RConn3 -- BUS-40/RConn3 -- Line-56/RConn3
  BUS-Load-30/RConn1 -- Load-30/LConn1
  BUS-Load-30/RConn2 -- Load-30/LConn2
  BUS-Load-30/RConn3 -- Load-30/LConn3
  BUS-SG-6/LConn1 -- SG-6/RConn1
  BUS-SG-6/LConn2 -- SG-6/RConn2
  BUS-SG-6/LConn3 -- SG-6/RConn3
  Line-59/LConn1 -- BUS-40/LConn1 -- Line-60/LConn1
  Line-59/LConn2 -- BUS-40/LConn2 -- Line-60/LConn2
  Line-59/LConn3 -- BUS-40/LConn3 -- Line-60/LConn3
  BUS-41/RConn1 -- Line-59/RConn1 -- BUS-Load-31/LConn1
  BUS-41/RConn2 -- Line-59/RConn2 -- BUS-Load-31/LConn2
  BUS-41/RConn3 -- Line-59/RConn3 -- BUS-Load-31/LConn3
  BUS-Load-31/RConn1 -- Load-31/LConn1
  BUS-Load-31/RConn2 -- Load-31/LConn2
  BUS-Load-31/RConn3 -- Load-31/LConn3
  BUS-41/LConn1 -- Line-61/LConn1
  BUS-41/LConn2 -- Line-61/LConn2
  BUS-41/LConn3 -- Line-61/LConn3
  Line-61/RConn1 -- BUS-Load-32/LConn1 -- BUS-42/RConn1 -- Line-60/RConn1
  Line-61/RConn2 -- BUS-Load-32/LConn2 -- BUS-42/RConn2 -- Line-60/RConn2
  Line-61/RConn3 -- BUS-Load-32/LConn3 -- BUS-42/RConn3 -- Line-60/RConn3
  BUS-Load-32/RConn1 -- Load-32/LConn1
  BUS-Load-32/RConn2 -- Load-32/LConn2
  BUS-Load-32/RConn3 -- Load-32/LConn3
  BUS-42/LConn1 -- Line-62/LConn1
  BUS-42/LConn2 -- Line-62/LConn2
  BUS-42/LConn3 -- Line-62/LConn3
  BUS-38/RConn1 -- Line-169/RConn1 -- Line-45/RConn1
  BUS-38/RConn2 -- Line-169/RConn2 -- Line-45/RConn2
  BUS-38/RConn3 -- Line-169/RConn3 -- Line-45/RConn3
  BUS-38/LConn1 -- Line-57/LConn1
  BUS-38/LConn2 -- Line-57/LConn2
  BUS-38/LConn3 -- Line-57/LConn3
  Line-45/LConn1 -- BUS-30/LConn1 -- Line-39/RConn1
  Line-45/LConn2 -- BUS-30/LConn2 -- Line-39/RConn2
  Line-45/LConn3 -- BUS-30/LConn3 -- Line-39/RConn3
  BUS-8/LConn1 -- Line-12/LConn1
  BUS-8/LConn2 -- Line-12/LConn2
  BUS-8/LConn3 -- Line-12/LConn3
  BUS-30/RConn1 -- Line-12/RConn1 -- Line-167/RConn1
  BUS-30/RConn2 -- Line-12/RConn2 -- Line-167/RConn2
  BUS-30/RConn3 -- Line-12/RConn3 -- Line-167/RConn3
  BUS-5/LConn1 -- Line-166/LConn1
  BUS-5/LConn2 -- Line-166/LConn2
  BUS-5/LConn3 -- Line-166/LConn3
  Line-166/RConn1 -- BUS-8/RConn1
  Line-166/RConn2 -- BUS-8/RConn2
  Line-166/RConn3 -- BUS-8/RConn3
  Line-8/LConn1 -- BUS-5/RConn1 -- Line-6/RConn1 -- Line-9/LConn1 -- Line-4/RConn1
  Line-8/LConn2 -- BUS-5/RConn2 -- Line-6/RConn2 -- Line-9/LConn2 -- Line-4/RConn2
  Line-8/LConn3 -- BUS-5/RConn3 -- Line-6/RConn3 -- Line-9/LConn3 -- Line-4/RConn3
  Line-8/RConn1 -- BUS-6/LConn1
  Line-8/RConn2 -- BUS-6/LConn2
  Line-8/RConn3 -- BUS-6/LConn3
  BUS-Load-5/LConn1 -- BUS-6/RConn1 -- Line-10/LConn1
  BUS-Load-5/LConn2 -- BUS-6/RConn2 -- Line-10/LConn2
  BUS-Load-5/LConn3 -- BUS-6/RConn3 -- Line-10/LConn3
  BUS-Load-5/RConn1 -- Load-5/LConn1
  BUS-Load-5/RConn2 -- Load-5/LConn2
  BUS-Load-5/RConn3 -- Load-5/LConn3
  Line-10/RConn1 -- BUS-7/LConn1
  Line-10/RConn2 -- BUS-7/LConn2
  Line-10/RConn3 -- BUS-7/LConn3
  BUS-Load-6/LConn1 -- BUS-7/RConn1 -- Line-11/LConn1
  BUS-Load-6/LConn2 -- BUS-7/RConn2 -- Line-11/LConn2
  BUS-Load-6/LConn3 -- BUS-7/RConn3 -- Line-11/LConn3
  BUS-Load-6/RConn1 -- Load-6/LConn1
  BUS-Load-6/RConn2 -- Load-6/LConn2
  BUS-Load-6/RConn3 -- Load-6/LConn3
  Line-11/RConn1 -- Line-15/LConn1 -- Line-13/RConn1 -- Line-16/LConn1 -- BUS-12/LConn1 -- Line-5/RConn1
  Line-11/RConn2 -- Line-15/LConn2 -- Line-13/RConn2 -- Line-16/LConn2 -- BUS-12/LConn2 -- Line-5/RConn2
  Line-11/RConn3 -- Line-15/LConn3 -- Line-13/RConn3 -- Line-16/LConn3 -- BUS-12/LConn3 -- Line-5/RConn3
  BUS-Load-8/LConn1 -- BUS-12/RConn1 -- BUS-SG-1/RConn1 -- Line-17/LConn1 -- Line-3/RConn1
  BUS-Load-8/LConn2 -- BUS-12/RConn2 -- BUS-SG-1/RConn2 -- Line-17/LConn2 -- Line-3/RConn2
  BUS-Load-8/LConn3 -- BUS-12/RConn3 -- BUS-SG-1/RConn3 -- Line-17/LConn3 -- Line-3/RConn3
  BUS-Load-8/RConn1 -- Load-8/LConn1
  BUS-Load-8/RConn2 -- Load-8/LConn2
  BUS-Load-8/RConn3 -- Load-8/LConn3
  BUS-SG-1/LConn1 -- SG-1/RConn1
  BUS-SG-1/LConn2 -- SG-1/RConn2
  BUS-SG-1/LConn3 -- SG-1/RConn3
  BUS-14/RConn1 -- Line-15/RConn1 -- BUS-Load-10/LConn1
  BUS-14/RConn2 -- Line-15/RConn2 -- BUS-Load-10/LConn2
  BUS-14/RConn3 -- Line-15/RConn3 -- BUS-Load-10/LConn3
  BUS-Load-10/RConn1 -- Load-10/LConn1
  BUS-Load-10/RConn2 -- Load-10/LConn2
  BUS-Load-10/RConn3 -- Load-10/LConn3
  BUS-14/LConn1 -- Line-19/LConn1
  BUS-14/LConn2 -- Line-19/LConn2
  BUS-14/LConn3 -- Line-19/LConn3
  Line-19/RConn1 -- BUS-Load-11/LConn1 -- BUS-15/RConn1 -- Line-18/RConn1
  Line-19/RConn2 -- BUS-Load-11/LConn2 -- BUS-15/RConn2 -- Line-18/RConn2
  Line-19/RConn3 -- BUS-Load-11/LConn3 -- BUS-15/RConn3 -- Line-18/RConn3
  BUS-Load-11/RConn1 -- Load-11/LConn1
  BUS-Load-11/RConn2 -- Load-11/LConn2
  BUS-Load-11/RConn3 -- Load-11/LConn3
  Line-20/LConn1 -- BUS-15/LConn1 -- Line-21/LConn1 -- Line-22/LConn1
  Line-20/LConn2 -- BUS-15/LConn2 -- Line-21/LConn2 -- Line-22/LConn2
  Line-20/LConn3 -- BUS-15/LConn3 -- Line-21/LConn3 -- Line-22/LConn3
  Line-22/RConn1 -- BUS-33/RConn1
  Line-22/RConn2 -- BUS-33/RConn2
  Line-22/RConn3 -- BUS-33/RConn3
  BUS-Load-25/LConn1 -- BUS-33/LConn1 -- Line-49/LConn1
  BUS-Load-25/LConn2 -- BUS-33/LConn2 -- Line-49/LConn2
  BUS-Load-25/LConn3 -- BUS-33/LConn3 -- Line-49/LConn3
  BUS-Load-25/RConn1 -- Load-25/LConn1
  BUS-Load-25/RConn2 -- Load-25/LConn2
  BUS-Load-25/RConn3 -- Load-25/LConn3
  BUS-13/LConn1 -- Line-18/LConn1
  BUS-13/LConn2 -- Line-18/LConn2
  BUS-13/LConn3 -- Line-18/LConn3
  BUS-Load-9/LConn1 -- BUS-13/RConn1 -- Line-14/RConn1
  BUS-Load-9/LConn2 -- BUS-13/RConn2 -- Line-14/RConn2
  BUS-Load-9/LConn3 -- BUS-13/RConn3 -- Line-14/RConn3
  BUS-Load-9/RConn1 -- Load-9/LConn1
  BUS-Load-9/RConn2 -- Load-9/LConn2
  BUS-Load-9/RConn3 -- Load-9/LConn3
  Line-14/LConn1 -- BUS-11/LConn1 -- Line-7/RConn1 -- Line-9/RConn1
  Line-14/LConn2 -- BUS-11/LConn2 -- Line-7/RConn2 -- Line-9/RConn2
  Line-14/LConn3 -- BUS-11/LConn3 -- Line-7/RConn3 -- Line-9/RConn3
  BUS-Load-7/LConn1 -- BUS-11/RConn1 -- Line-13/LConn1
  BUS-Load-7/LConn2 -- BUS-11/RConn2 -- Line-13/LConn2
  BUS-Load-7/LConn3 -- BUS-11/RConn3 -- Line-13/LConn3
  BUS-Load-7/RConn1 -- Load-7/LConn1
  BUS-Load-7/RConn2 -- Load-7/LConn2
  BUS-Load-7/RConn3 -- Load-7/LConn3
  BUS-4/RConn1 -- Line-7/LConn1
  BUS-4/RConn2 -- Line-7/LConn2
  BUS-4/RConn3 -- Line-7/LConn3
  BUS-Load-4/LConn1 -- BUS-4/LConn1 -- Line-6/LConn1
  BUS-Load-4/LConn2 -- BUS-4/LConn2 -- Line-6/LConn2
  BUS-Load-4/LConn3 -- BUS-4/LConn3 -- Line-6/LConn3
  BUS-Load-4/RConn1 -- Load-4/LConn1
  BUS-Load-4/RConn2 -- Load-4/LConn2
  BUS-Load-4/RConn3 -- Load-4/LConn3
  BUS-16/RConn1 -- Line-16/RConn1 -- BUS-Load-12/LConn1
  BUS-16/RConn2 -- Line-16/RConn2 -- BUS-Load-12/LConn2
  BUS-16/RConn3 -- Line-16/RConn3 -- BUS-Load-12/LConn3
  BUS-Load-12/RConn1 -- Load-12/LConn1
  BUS-Load-12/RConn2 -- Load-12/LConn2
  BUS-Load-12/RConn3 -- Load-12/LConn3
  BUS-16/LConn1 -- Line-23/LConn1
  BUS-16/LConn2 -- Line-23/LConn2
  BUS-16/LConn3 -- Line-23/LConn3
  Line-17/RConn1 -- BUS-117/LConn1
  Line-17/RConn2 -- BUS-117/LConn2
  Line-17/RConn3 -- BUS-117/LConn3
  BUS-117/RConn1 -- BUS-Load-90/LConn1
  BUS-117/RConn2 -- BUS-Load-90/LConn2
  BUS-117/RConn3 -- BUS-Load-90/LConn3
  BUS-Load-90/RConn1 -- Load-90/LConn1
  BUS-Load-90/RConn2 -- Load-90/LConn2
  BUS-Load-90/RConn3 -- Load-90/LConn3
  Line-3/LConn1 -- BUS-2/LConn1 -- Line-1/RConn1
  Line-3/LConn2 -- BUS-2/LConn2 -- Line-1/RConn2
  Line-3/LConn3 -- BUS-2/LConn3 -- Line-1/RConn3
  BUS-2/RConn1 -- BUS-Load-2/LConn1
  BUS-2/RConn2 -- BUS-Load-2/LConn2
  BUS-2/RConn3 -- BUS-Load-2/LConn3
  BUS-Load-2/RConn1 -- Load-2/LConn1
  BUS-Load-2/RConn2 -- Load-2/LConn2
  BUS-Load-2/RConn3 -- Load-2/LConn3
  Line-1/LConn1 -- BUS-1/RConn1 -- BUS-Load-1/LConn1
  Line-1/LConn2 -- BUS-1/RConn2 -- BUS-Load-1/LConn2
  Line-1/LConn3 -- BUS-1/RConn3 -- BUS-Load-1/LConn3
  BUS-Load-1/RConn1 -- Load-1/LConn1
  BUS-Load-1/RConn2 -- Load-1/LConn2
  BUS-Load-1/RConn3 -- Load-1/LConn3
  BUS-1/LConn1 -- Line-2/LConn1
  BUS-1/LConn2 -- Line-2/LConn2
  BUS-1/LConn3 -- Line-2/LConn3
  Line-2/RConn1 -- BUS-Load-3/LConn1 -- BUS-3/RConn1 -- Line-5/LConn1
  Line-2/RConn2 -- BUS-Load-3/LConn2 -- BUS-3/RConn2 -- Line-5/LConn2
  Line-2/RConn3 -- BUS-Load-3/LConn3 -- BUS-3/RConn3 -- Line-5/LConn3
  BUS-Load-3/RConn1 -- Load-3/LConn1
  BUS-Load-3/RConn2 -- Load-3/LConn2
  BUS-Load-3/RConn3 -- Load-3/LConn3
  BUS-3/LConn1 -- Line-4/LConn1
  BUS-3/LConn2 -- Line-4/LConn2
  BUS-3/LConn3 -- Line-4/LConn3
  BUS-26/RConn1 -- Line-39/LConn1
  BUS-26/RConn2 -- Line-39/LConn2
  BUS-26/RConn3 -- Line-39/LConn3
  Line-168/RConn1 -- BUS-26/LConn1
  Line-168/RConn2 -- BUS-26/LConn2
  Line-168/RConn3 -- BUS-26/LConn3
  Line-51/LConn1 -- BUS-34/LConn1 -- Line-52/LConn1
  Line-51/LConn2 -- BUS-34/LConn2 -- Line-52/LConn2
  Line-51/LConn3 -- BUS-34/LConn3 -- Line-52/LConn3
  BUS-43/RConn1 -- Line-52/RConn1 -- BUS-Load-33/LConn1
  BUS-43/RConn2 -- Line-52/RConn2 -- BUS-Load-33/LConn2
  BUS-43/RConn3 -- Line-52/RConn3 -- BUS-Load-33/LConn3
  BUS-Load-33/RConn1 -- Load-33/LConn1
  BUS-Load-33/RConn2 -- Load-33/LConn2
  BUS-Load-33/RConn3 -- Load-33/LConn3
  BUS-43/LConn1 -- Line-63/LConn1
  BUS-43/LConn2 -- Line-63/LConn2
  BUS-43/LConn3 -- Line-63/LConn3
  BUS-44/RConn1 -- Line-63/RConn1 -- BUS-Load-34/LConn1
  BUS-44/RConn2 -- Line-63/RConn2 -- BUS-Load-34/LConn2
  BUS-44/RConn3 -- Line-63/RConn3 -- BUS-Load-34/LConn3
  BUS-Load-34/RConn1 -- Load-34/LConn1
  BUS-Load-34/RConn2 -- Load-34/LConn2
  BUS-Load-34/RConn3 -- Load-34/LConn3
  BUS-44/LConn1 -- Line-64/LConn1
  BUS-44/LConn2 -- Line-64/LConn2
  BUS-44/LConn3 -- Line-64/LConn3
  BUS-45/RConn1 -- Line-64/RConn1 -- BUS-Load-35/LConn1
  BUS-45/RConn2 -- Line-64/RConn2 -- BUS-Load-35/LConn2
  BUS-45/RConn3 -- Line-64/RConn3 -- BUS-Load-35/LConn3
  BUS-Load-35/RConn1 -- Load-35/LConn1
  BUS-Load-35/RConn2 -- Load-35/LConn2
  BUS-Load-35/RConn3 -- Load-35/LConn3
  Line-65/LConn1 -- BUS-45/LConn1 -- Line-66/LConn1
  Line-65/LConn2 -- BUS-45/LConn2 -- Line-66/LConn2
  Line-65/LConn3 -- BUS-45/LConn3 -- Line-66/LConn3
  BUS-46/RConn1 -- Line-65/RConn1 -- BUS-Load-36/LConn1
  BUS-46/RConn2 -- Line-65/RConn2 -- BUS-Load-36/LConn2
  BUS-46/RConn3 -- Line-65/RConn3 -- BUS-Load-36/LConn3
  BUS-Load-36/RConn1 -- Load-36/LConn1
  BUS-Load-36/RConn2 -- Load-36/LConn2
  BUS-Load-36/RConn3 -- Load-36/LConn3
  BUS-SG-7/RConn1 -- BUS-46/LConn1 -- Line-67/LConn1 -- Line-68/LConn1
  BUS-SG-7/RConn2 -- BUS-46/LConn2 -- Line-67/LConn2 -- Line-68/LConn2
  BUS-SG-7/RConn3 -- BUS-46/LConn3 -- Line-67/LConn3 -- Line-68/LConn3
  BUS-SG-7/LConn1 -- SG-7/RConn1
  BUS-SG-7/LConn2 -- SG-7/RConn2
  BUS-SG-7/LConn3 -- SG-7/RConn3
  BUS-47/RConn1 -- Line-67/RConn1 -- BUS-Load-37/LConn1
  BUS-47/RConn2 -- Line-67/RConn2 -- BUS-Load-37/LConn2
  BUS-47/RConn3 -- Line-67/RConn3 -- BUS-Load-37/LConn3
  BUS-Load-37/RConn1 -- Load-37/LConn1
  BUS-Load-37/RConn2 -- Load-37/LConn2
  BUS-Load-37/RConn3 -- Load-37/LConn3
  Line-69/LConn1 -- BUS-47/LConn1 -- Line-70/LConn1
  Line-69/LConn2 -- BUS-47/LConn2 -- Line-70/LConn2
  Line-69/LConn3 -- BUS-47/LConn3 -- Line-70/LConn3
  BUS-48/RConn1 -- Line-68/RConn1 -- Line-71/LConn1
  BUS-48/RConn2 -- Line-68/RConn2 -- Line-71/LConn2
  BUS-48/RConn3 -- Line-68/RConn3 -- Line-71/LConn3
  BUS-48/LConn1 -- BUS-Load-38/LConn1
  BUS-48/LConn2 -- BUS-Load-38/LConn2
  BUS-48/LConn3 -- BUS-Load-38/LConn3
  BUS-Load-38/RConn1 -- Load-38/LConn1
  BUS-Load-38/RConn2 -- Load-38/LConn2
  BUS-Load-38/RConn3 -- Load-38/LConn3
  BUS-114/LConn1 -- Line-48/RConn1 -- Line-165/LConn1
  BUS-114/LConn2 -- Line-48/RConn2 -- Line-165/LConn2
  BUS-114/LConn3 -- Line-48/RConn3 -- Line-165/LConn3
  BUS-114/RConn1 -- BUS-Load-88/LConn1
  BUS-114/RConn2 -- BUS-Load-88/LConn2
  BUS-114/RConn3 -- BUS-Load-88/LConn3
  BUS-Load-88/RConn1 -- Load-88/LConn1
  BUS-Load-88/RConn2 -- Load-88/LConn2
  BUS-Load-88/RConn3 -- Load-88/LConn3
  BUS-115/RConn1 -- Line-165/RConn1 -- BUS-Load-89/LConn1
  BUS-115/RConn2 -- Line-165/RConn2 -- BUS-Load-89/LConn2
  BUS-115/RConn3 -- Line-165/RConn3 -- BUS-Load-89/LConn3
  BUS-Load-89/RConn1 -- Load-89/LConn1
  BUS-Load-89/RConn2 -- Load-89/LConn2
  BUS-Load-89/RConn3 -- Load-89/LConn3
  Line-42/RConn1 -- BUS-115/LConn1
  Line-42/RConn2 -- BUS-115/LConn2
  Line-42/RConn3 -- BUS-115/LConn3
  BUS-71/LConn1 -- Line-109/LConn1
  BUS-71/LConn2 -- Line-109/LConn2
  BUS-71/LConn3 -- Line-109/LConn3
  Line-109/RConn1 -- BUS-73/RConn1
  Line-109/RConn2 -- BUS-73/RConn2
  Line-109/RConn3 -- BUS-73/RConn3
  BUS-73/LConn1 -- BUS-SG-14/RConn1
  BUS-73/LConn2 -- BUS-SG-14/RConn2
  BUS-73/LConn3 -- BUS-SG-14/RConn3
  BUS-SG-14/LConn1 -- SG-14/RConn1
  BUS-SG-14/LConn2 -- SG-14/RConn2
  BUS-SG-14/LConn3 -- SG-14/RConn3
  Line-106/RConn1 -- BUS-74/RConn1
  Line-106/RConn2 -- BUS-74/RConn2
  Line-106/RConn3 -- BUS-74/RConn3
  BUS-Load-55/LConn1 -- BUS-74/LConn1 -- Line-110/LConn1
  BUS-Load-55/LConn2 -- BUS-74/LConn2 -- Line-110/LConn2
  BUS-Load-55/LConn3 -- BUS-74/LConn3 -- Line-110/LConn3
  BUS-Load-55/RConn1 -- Load-55/LConn1
  BUS-Load-55/RConn2 -- Load-55/LConn2
  BUS-Load-55/RConn3 -- Load-55/LConn3
  Line-110/RConn1 -- Line-103/RConn1 -- BUS-75/RConn1 -- Line-107/RConn1
  Line-110/RConn2 -- Line-103/RConn2 -- BUS-75/RConn2 -- Line-107/RConn2
  Line-110/RConn3 -- Line-103/RConn3 -- BUS-75/RConn3 -- Line-107/RConn3
  BUS-Load-56/LConn1 -- BUS-75/LConn1 -- Line-111/LConn1 -- Line-112/LConn1
  BUS-Load-56/LConn2 -- BUS-75/LConn2 -- Line-111/LConn2 -- Line-112/LConn2
  BUS-Load-56/LConn3 -- BUS-75/LConn3 -- Line-111/LConn3 -- Line-112/LConn3
  BUS-Load-56/RConn1 -- Load-56/LConn1
  BUS-Load-56/RConn2 -- Load-56/LConn2
  BUS-Load-56/RConn3 -- Load-56/LConn3
  Line-112/RConn1 -- BUS-118/RConn1
  Line-112/RConn2 -- BUS-118/RConn2
  Line-112/RConn3 -- BUS-118/RConn3
  BUS-Load-91/LConn1 -- BUS-118/LConn1 -- Line-114/RConn1
  BUS-Load-91/LConn2 -- BUS-118/LConn2 -- Line-114/RConn2
  BUS-Load-91/LConn3 -- BUS-118/LConn3 -- Line-114/RConn3
  BUS-Load-91/RConn1 -- Load-91/LConn1
  BUS-Load-91/RConn2 -- Load-91/LConn2
  BUS-Load-91/RConn3 -- Load-91/LConn3
  Line-114/LConn1 -- BUS-76/RConn1 -- Line-113/LConn1
  Line-114/LConn2 -- BUS-76/RConn2 -- Line-113/LConn2
  Line-114/LConn3 -- BUS-76/RConn3 -- Line-113/LConn3
  BUS-Load-57/LConn1 -- BUS-76/LConn1 -- BUS-SG-15/RConn1 -- BUS-VSC-5/RConn1 -- BUS-VSC-15/RConn1
  BUS-Load-57/LConn2 -- BUS-76/LConn2 -- BUS-SG-15/RConn2 -- BUS-VSC-5/RConn2 -- BUS-VSC-15/RConn2
  BUS-Load-57/LConn3 -- BUS-76/LConn3 -- BUS-SG-15/RConn3 -- BUS-VSC-5/RConn3 -- BUS-VSC-15/RConn3
  BUS-Load-57/RConn1 -- Load-57/LConn1
  BUS-Load-57/RConn2 -- Load-57/LConn2
  BUS-Load-57/RConn3 -- Load-57/LConn3
  BUS-SG-15/LConn1 -- SG-15/RConn1
  BUS-SG-15/LConn2 -- SG-15/RConn2
  BUS-SG-15/LConn3 -- SG-15/RConn3
  BUS-VSC-5/LConn1 -- VSC-5/RConn1
  BUS-VSC-5/LConn2 -- VSC-5/RConn2
  BUS-VSC-5/LConn3 -- VSC-5/RConn3
  BUS-VSC-15/LConn1 -- VSC-15/RConn1
  BUS-VSC-15/LConn2 -- VSC-15/RConn2
  BUS-VSC-15/LConn3 -- VSC-15/RConn3
  BUS-64/RConn1 -- Line-98/LConn1
  BUS-64/RConn2 -- Line-98/LConn2
  BUS-64/RConn3 -- Line-98/LConn3
  BUS-63/RConn1 -- Line-97/LConn1
  BUS-63/RConn2 -- Line-97/LConn2
  BUS-63/RConn3 -- Line-97/LConn3
  BUS-64/LConn1 -- Line-97/RConn1 -- Line-171/RConn1
  BUS-64/LConn2 -- Line-97/RConn2 -- Line-171/RConn2
  BUS-64/LConn3 -- Line-97/RConn3 -- Line-171/RConn3
  Line-170/RConn1 -- BUS-63/LConn1
  Line-170/RConn2 -- BUS-63/LConn2
  Line-170/RConn3 -- BUS-63/LConn3
